simulink model "uz_pmsm_model_6LUT_pd"  (R2023b)
settings: Solver=FixedStepAuto  StartTime=0.0  StopTime=0.05  RelTol=1e-3
PreLoadFcn:
  | uz_pmsm_model_init_parameter
PostLoadFcn:
  | % Import the data from Excel for a lookup table
  | FluxMapData = readtable('C:\Users\Philipp\ultrazohm\ultrazohm_sw\ip_cores\uz_pmsm_model\FluxMapData_2023-05-26_13-07-57.csv');
  | % Row indices for lookup table
  | d_current_in_d_axis = FluxMapData(8:27,1:end);
  | % Column indices for lookup table
  | q_current_in_d_axis = FluxMapData(29:48,1:end);
  | % Output values for lookup table
  | d_Flux_d_axis = FluxMapData(50:69,1:end);
values from neighbouring files (symbols this model uses):
  ad1 = 7.2940    (= 7.294)    [LUT_approx_methode1_u_2b.m]    (also in LUT_approx_methode1_u_2b_alt.m; LUT_approx_methode2a.m = ad_1(1); LUT_approx_methode_2a_FEM.m = ad_1(1); LUT_approx_new.m = ad_1(1))
  ad2 = 0.0001    [LUT_approx_methode1_u_2b.m]    (also in LUT_approx_methode1_u_2b_alt.m; LUT_approx_methode2a.m = ad_1(2); LUT_approx_methode_2a_FEM.m = ad_1(2); LUT_approx_new.m = ad_1(2))
  ad3 = -15.5992    [LUT_approx_methode1_u_2b.m]    (also in LUT_approx_methode1_u_2b_alt.m; LUT_approx_methode2a.m = ad_1(3); LUT_approx_methode_2a_FEM.m = ad_1(3); LUT_approx_new.m = ad_1(3))
  ad4 = -186.4725    [LUT_approx_methode1_u_2b.m]    (also in LUT_approx_methode1_u_2b_alt.m; LUT_approx_methode2a.m = ad_3_6(1); LUT_approx_methode_2a_FEM.m = ad_3_6(1); LUT_approx_new.m = ad_3_6(1))
  ad5 = 187.4853    [LUT_approx_methode1_u_2b.m]    (also in LUT_approx_methode1_u_2b_alt.m; LUT_approx_methode2a.m = ad_3_6(2); LUT_approx_methode_2a_FEM.m = ad_3_6(2); LUT_approx_new.m = ad_3_6(2))
  ad6 = 0.0000    (= 0)    [LUT_approx_methode1_u_2b.m]    (also in LUT_approx_methode1_u_2b_alt.m; LUT_approx_methode2a.m = ad_3_6(3); LUT_approx_methode_2a_FEM.m = ad_3_6(3); LUT_approx_new.m = ad_3_6(3))
  aq1 = 0.0041    [LUT_approx_methode1_u_2b.m]    (also in LUT_approx_methode1_u_2b_alt.m; LUT_approx_methode2a.m = aq_1(1); LUT_approx_methode_2a_FEM.m = aq_1(1); LUT_approx_new.m = aq_1(1))
  aq2 = 0.2092    [LUT_approx_methode1_u_2b.m]    (also in LUT_approx_methode1_u_2b_alt.m; LUT_approx_methode2a.m = aq_1(2); LUT_approx_methode_2a_FEM.m = aq_1(2); LUT_approx_new.m = aq_1(2))
  aq3 = 0.0010    (= 0.001)    [LUT_approx_methode1_u_2b.m]    (also in LUT_approx_methode1_u_2b_alt.m; LUT_approx_methode2a.m = aq_1(3); LUT_approx_methode_2a_FEM.m = aq_1(3); LUT_approx_new.m = aq_1(3))
  aq4 = 28.4940    (= 28.494)    [LUT_approx_methode1_u_2b.m]    (also in LUT_approx_methode1_u_2b_alt.m; LUT_approx_methode2a.m = aq_3_6(1); LUT_approx_methode_2a_FEM.m = aq_3_6(1); LUT_approx_new.m = aq_3_6(1))
  aq5 = -24.2348    [LUT_approx_methode1_u_2b.m]    (also in LUT_approx_methode1_u_2b_alt.m; LUT_approx_methode2a.m = aq_3_6(2); LUT_approx_methode_2a_FEM.m = aq_3_6(2); LUT_approx_new.m = aq_3_6(2))
  aq6 = 0.0405    [LUT_approx_methode1_u_2b.m]    (also in LUT_approx_methode1_u_2b_alt.m; LUT_approx_methode2a.m = aq_3_6(3); LUT_approx_methode_2a_FEM.m = aq_3_6(3); LUT_approx_new.m = aq_3_6(3))
  d_current_d_Flux = FluxMapData{1,1:20}    [uz_pmsm_model_6LUT_pd_init_parameter.m]
  d_current_q_Flux = FluxMapData{66,1:20}    [uz_pmsm_model_6LUT_pd_init_parameter.m]
  entkopplung_dynamic = false    [uz_pmsm_model_6LUT_pd_init_parameter.m]
  entkopplung_linear = true    [uz_pmsm_model_6LUT_pd_init_parameter.m]
  entkopplung_static = false    [uz_pmsm_model_6LUT_pd_init_parameter.m]
  Fid1_Giq1 = ((1/2).*(aq3-aq6).*((q_current_set).^2))+((aq1./aq2).*log(cosh(aq2.*q_current_set)))-((aq4/aq5).*log(cosh(aq5.*q_current_set)))    [LUT_approx_methode2a.m]    (also in LUT_approx_methode_2a_FEM.m = (1/2).*(aq3-aq6).*((q_current_set).^2)+((aq1./aq2).*log(cosh; LUT_approx_new.m = (1/2)*(aq3-aq6)*((q_current_set).^2)+((aq1/aq2)*log(cosh(aq2; LUT_approximation_fitting.m = (1/2)*(aq3-aq6)*((iq1)^2)+((aq1/aq2)*log(cosh(aq2*iq1)))-((a)
  Fid2_Giq2 = ((ad1./ad2).*(log(cosh(ad2.*(d_current_set-ad3))))) - ((ad4./ad5).*(log(cosh(ad5.*(d_current_set-ad6)))))    [LUT_approx_methode2a.m]    (also in LUT_approx_methode_2a_FEM.m = ((ad1./ad2).*(log(cosh(ad2.*(d_current_set-ad3))))) - (((ad1)
  Flux_d = FluxMapData{43:62,1:20}'*(1e-3)    [uz_pmsm_model_6LUT_pd_init_parameter.m]
  Flux_q = FluxMapData{108:127,1:20}'*(1e-3)    [uz_pmsm_model_6LUT_pd_init_parameter.m]
  friction_coefficient = 0.001    [uz_pmsm_model_6LUT_pd_init_parameter.m]
  inertia = 0.000084    (= 8.4e-05)    [uz_pmsm_model_6LUT_pd_init_parameter.m]
  L_d = 0.00045    [uz_pmsm_model_6LUT_pd_init_parameter.m]
  L_q = 0.002    [uz_pmsm_model_6LUT_pd_init_parameter.m]
  parameter_nachfuerung = true    [uz_pmsm_model_6LUT_pd_init_parameter.m]
  polepair = 4    [uz_pmsm_model_6LUT_pd_init_parameter.m]
  praediktion_entkopplung_nonlinear = true    [uz_pmsm_model_6LUT_pd_init_parameter.m]
  psi_pm = 0.0194    [uz_pmsm_model_6LUT_pd_init_parameter.m]
  q_current_d_Flux = FluxMapData{22:41,1}    [uz_pmsm_model_6LUT_pd_init_parameter.m]
  q_current_q_Flux = FluxMapData{87:106,1}    [uz_pmsm_model_6LUT_pd_init_parameter.m]
  R_1 = 0.3    [uz_pmsm_model_6LUT_pd_init_parameter.m]
  simulate_mechanical = false    [uz_pmsm_model_6LUT_pd_init_parameter.m]
  simulate_nonlinear_modell = true    [uz_pmsm_model_6LUT_pd_init_parameter.m]
  simulate_open_loop = false    [uz_pmsm_model_6LUT_pd_init_parameter.m]
  static_friction_torque = 0.01    [uz_pmsm_model_6LUT_pd_init_parameter.m]
  tau_sum = 2*ts_regler    (= 8e-05)    [uz_pmsm_model_6LUT_pd_init_parameter.m]
  ts = 1/5e5    (= 2e-06)    [uz_pmsm_model_6LUT_pd_init_parameter.m]
  ts_regler = 1/25e3    (= 4e-05)    [uz_pmsm_model_6LUT_pd_init_parameter.m]
undefined symbols (not defined in the file or in its folder): Ki_Bo_d, Ki_Bo_q, Kp_Bo_d, Kp_Bo_q, Ldq
libraries: slpidlib x2
(part 1 of 2)
settings Model: DataTypeOverride=Off  Creator=ts  LastModifiedBy=Philipp
settings SolverCC: AlgebraicLoopSolver=TrustRegion  AutoInsertRateTranBlk=on
settings DataIOCC: LimitDataPoints=on  SaveOutput=off  SaveTime=off
settings OptimizationCC: BlockReduction=off  ConditionallyExecuteInputs=off  DefaultParameterBehavior=Inlined  LifeSpan=inf
settings DebuggingCC: AlgebraicLoopMsg=error  SingleTaskRateTransMsg=error  UnconnectedInputMsg=warning  UnconnectedOutputMsg=warning  UnconnectedLineMsg=warning  AllowSymbolicDim=off  StrictBusMsg=ErrorOnBusTreatedAsVector  SFUnexpectedBacktrackingDiag=warning  SFNoUnconditionalDefaultTransitionDiag=warning  SFExecutionAtInitializationDiag=none  ArithmeticOperatorsInVariantConditions=warning
settings HardwareCC: ProdBitPerPointer=32  ProdBitPerSizeT=32  ProdBitPerPtrDiffT=32  ProdLargestAtomicFloat=None  ProdIntDivRoundTo=Undefined  ProdEndianess=Unspecified  ProdWordSize=32  ProdHWDeviceType=ASIC/FPGA->ASIC/FPGA  ProdEqTarget=off
settings ModelReferenceCC: EnableRefExpFcnMdlSchedulingChecks=on
settings SFSimCC: SimUseLocalCustomCode=off  CustomCodeUndefinedFunction=UseInterfaceOnly
settings RTWCC: RTWUseLocalCustomCode=off  DLArmComputeVersion=19.05
settings CodeAppCC: StateflowObjectComments=on
settings GRTTargetCC: TargetLangStandard=C89/C90 (ANSI)
settings ConfigComp: CovScope=ReferencedModels  CovMetricSettings=dw  CovSaveCumulativeToWorkspaceVar=on  CovSaveSingleToWorkspaceVar=on  CovExternalEMLEnable=off  CovSFcnEnable=off

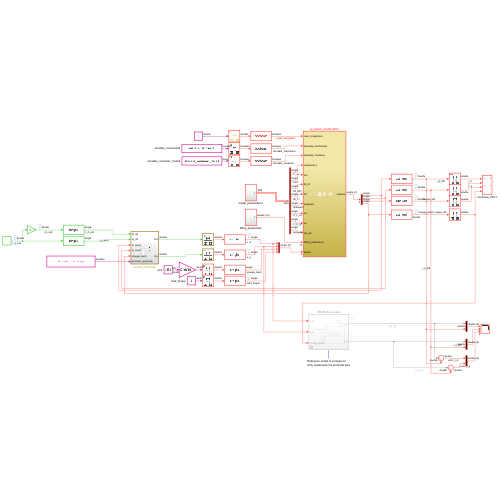
[thumbnail: Simulink's stored preview of the top-level diagram]
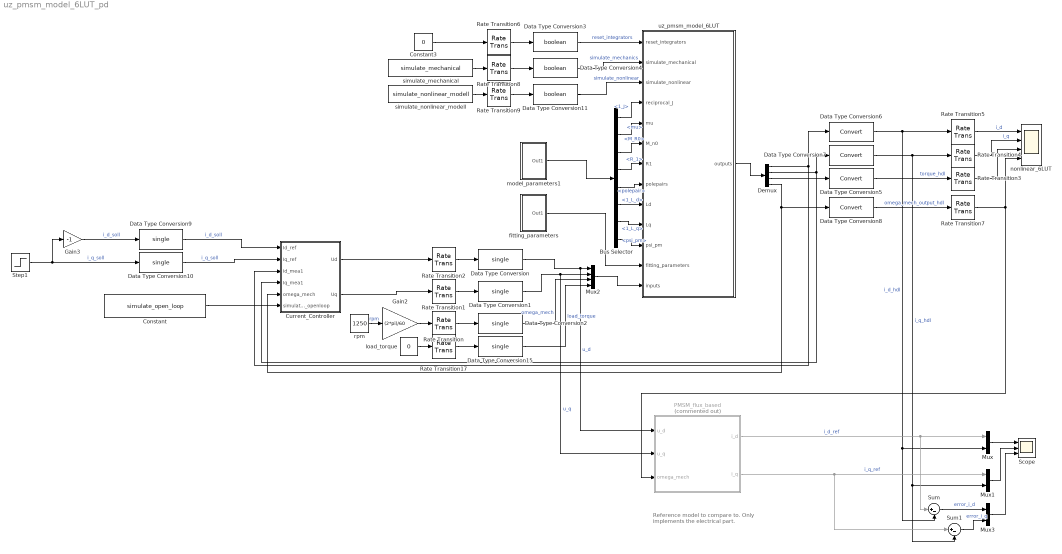
== system uz_pmsm_model_6LUT_pd ==
  note: Reference model to compare to.
      | Only implements the electrical part.
  Bus Selector : BusSelector  OutputSignals=1_J,mu,M_R0,R_1,polepair,1_L_d,1_L_q,psi_pm
  Constant : Constant  Value=simulate_open_loop
  Constant3 : Constant  Value=0
  Current_Controller : Subsystem
  Data Type Conversion{,1..2,9..10,15} (6 alike) : DataTypeConversion  OutDataTypeStr=single  SaturateOnIntegerOverflow=off  RndMeth=Floor
  Data Type Conversion11 : DataTypeConversion  OutDataTypeStr=boolean  SaturateOnIntegerOverflow=off  RndMeth=Floor
  Data Type Conversion3 : DataTypeConversion  OutDataTypeStr=boolean  SaturateOnIntegerOverflow=off  RndMeth=Floor
  Data Type Conversion4 : DataTypeConversion  OutDataTypeStr=boolean  SaturateOnIntegerOverflow=off  RndMeth=Floor
  Data Type Conversion{5..8} (4 alike) : DataTypeConversion  SaturateOnIntegerOverflow=off  RndMeth=Floor
  Demux : Demux
  Gain2 : Gain  Gain=(2*pi)/60
  Gain3 : Gain  Gain=-1
  Mux : Mux  Inputs=2
  Mux1 : Mux  Inputs=2
  Mux2 : Mux
  Mux3 : Mux  Inputs=2
  PMSM_flux_based : Subsystem  Commented=on
  Rate Transition{,1..2,6,8..9,17} (7 alike) : RateTransition  OutPortSampleTime=ts
  Rate Transition{3..5,7} (4 alike) : RateTransition
  Scope : Scope  NumInputPorts=3
  Step1 : Step  Time=0.025  After=5
  Sum : Sum  Inputs=|+-
  Sum1 : Sum  Inputs=|+-
  fitting_parameters : Subsystem
  load_torque : Constant  Value=0
  model_parameters1 : Subsystem
  nonlinear_6LUT : Scope  NumInputPorts=4
  rpm : Constant  Value=1250
  simulate_mechanical : Constant  Value=simulate_mechanical
  simulate_nonlinear_modell : Constant  Value=simulate_nonlinear_modell
  uz_pmsm_model_6LUT : Subsystem  TreatAsAtomicUnit=on
  wires:
  Rate Transition/1 -> Data Type Conversion2/1
  Rate Transition1/1 -> Data Type Conversion1/1
  Rate Transition2/1 -> Data Type Conversion/1
  Data Type Conversion6/1 -> Mux/2, Sum/2, Rate Transition5/1  "i_d_hdl"
  Data Type Conversion7/1 -> Rate Transition4/1, Mux1/2, Sum1/2  "i_q_hdl"
  Data Type Conversion5/1 -> Rate Transition3/1  "torque_hdl"
  Rate Transition4/1 -> nonlinear_6LUT/2  "i_q"
  Rate Transition5/1 -> nonlinear_6LUT/1  "i_d"
  Rate Transition3/1 -> nonlinear_6LUT/3
  Rate Transition6/1 -> Data Type Conversion3/1
  Constant3/1 -> Rate Transition6/1
  Rate Transition8/1 -> Data Type Conversion4/1
  simulate_mechanical/1 -> Rate Transition8/1
  Data Type Conversion3/1 -> uz_pmsm_model_6LUT/1(reset_integrators)  "reset_integrators"
  Data Type Conversion4/1 -> uz_pmsm_model_6LUT/2(simulate_mechanical)  "simulate_mechanics"
  load_torque/1 -> Rate Transition17/1
  Rate Transition17/1 -> Data Type Conversion15/1
  Mux/1 -> Scope/1
  Mux1/1 -> Scope/2
  PMSM_flux_based/2(i_q) -> Mux1/1, Sum1/1  "i_q_ref"
  PMSM_flux_based/1(i_d) -> Mux/1, Sum/1  "i_d_ref"
  Data Type Conversion8/1 -> Rate Transition7/1  "omega_mech_output_hdl"
  Rate Transition7/1 -> PMSM_flux_based/3(omega_mech), nonlinear_6LUT/4
  Bus Selector/1 -> uz_pmsm_model_6LUT/4(reciprocal_J)  "<1_J>"
  Bus Selector/2 -> uz_pmsm_model_6LUT/5(mu)  "<mu>"
  Bus Selector/3 -> uz_pmsm_model_6LUT/6(M_n0)  "<M_R0>"
  Bus Selector/4 -> uz_pmsm_model_6LUT/7(R1)  "<R_1>"
  Bus Selector/5 -> uz_pmsm_model_6LUT/8(polepairs)  "<polepair>"
  model_parameters1/1(Out1) -> Bus Selector/1
  Sum/1 -> Mux3/1  "error_i_d"
  Sum1/1 -> Mux3/2  "error_i_q"
  Mux3/1 -> Scope/3
  Step1/1 -> Gain3/1, Data Type Conversion10/1  "i_q_soll"
  Demux/3 -> Data Type Conversion5/1
  Gain3/1 -> Data Type Conversion9/1  "i_d_soll"
  Demux/1 -> Current_Controller/3(Id_mea1), Data Type Conversion6/1
  Demux/4 -> Current_Controller/5(omega_mech), Data Type Conversion8/1
  Demux/2 -> Current_Controller/4(Iq_mea1), Data Type Conversion7/1
  Data Type Conversion/1 -> PMSM_flux_based/1(u_d), Mux2/1  "u_d"
  Data Type Conversion1/1 -> PMSM_flux_based/2(u_q), Mux2/2  "u_q"
  Data Type Conversion15/1 -> Mux2/4  "load_torque"
  Data Type Conversion2/1 -> Mux2/3  "omega_mech"
  Mux2/1 -> uz_pmsm_model_6LUT/13(inputs)
  uz_pmsm_model_6LUT/1(outputs) -> Demux/1
  Data Type Conversion9/1 -> Current_Controller/1(Id_ref)  "i_d_soll"
  Data Type Conversion10/1 -> Current_Controller/2(Iq_ref)  "i_q_soll"
  Current_Controller/1(Ud) -> Rate Transition2/1
  Current_Controller/2(Uq) -> Rate Transition1/1
  Gain2/1 -> Rate Transition/1
  Constant/1 -> Current_Controller/6(simulate_openloop)
  rpm/1 -> Gain2/1  "rpm"
  simulate_nonlinear_modell/1 -> Rate Transition9/1
  Rate Transition9/1 -> Data Type Conversion11/1
  Bus Selector/6 -> uz_pmsm_model_6LUT/9(Ld)  "<1_L_d>"
  Bus Selector/7 -> uz_pmsm_model_6LUT/10(Lq)  "<1_L_q>"
  Bus Selector/8 -> uz_pmsm_model_6LUT/11(psi_pm)  "<psi_pm>"
  Data Type Conversion11/1 -> uz_pmsm_model_6LUT/3(simulate_nonlinear)  "simulate_nonlinear"
  fitting_parameters/1(Out1) -> uz_pmsm_model_6LUT/12(fitting_parameters)

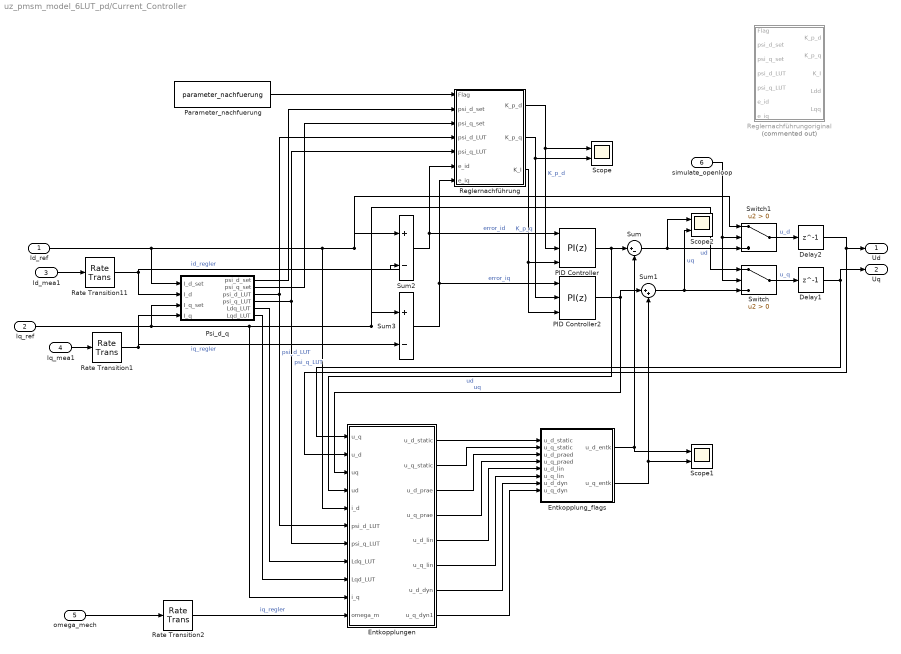
== system uz_pmsm_model_6LUT_pd/Current_Controller ==
  Id_ref : Inport
  Iq_ref : Inport  Port=2
  Id_mea1 : Inport  Port=3
  Iq_mea1 : Inport  Port=4
  omega_mech : Inport  Port=5
  simulate_openloop : Inport  Port=6
  Delay1 : Delay  DelayLength=1
  Delay2 : Delay  DelayLength=1
  Entkopplung_flags : Subsystem
  Entkopplungen : Subsystem
  PID Controller : slpidlib/PID Controller  Controller=PI  Form=Parallel  TimeDomain=Discrete-time  UseExternalTs=off  SampleTime=-1  IntegratorMethod=Forward Euler  FilterMethod=Forward Euler  ControllerParametersSource=external  P=Kp_Bo_d  I=Ki_Bo_d  UseKiTs=off  D=0  N=100  UseFilter=on  TunerSelectOption=Transfer Function Based (PID Tuner App)  InitialConditionSource=internal  InitialConditionForIntegrator=0  InitialConditionForFilter=0  DifferentiatorICPrevScaledInput=0  ExternalReset=none  TrackingMode=off  Kt=1  LimitOutput=off  SatLimitsSource=internal  UpperSaturationLimit=48  LowerSaturationLimit=-48  LinearizeAsGain=off  AntiWindupMode=clamping  Kb=1  LimitIntegrator=off  UpperIntegratorSaturationLimit=48  LowerIntegratorSaturationLimit=-48  POutMin=[]  POutMax=[]  IOutMin=[]  IOutMax=[]  DOutMin=[]  DOutMax=[]  NOutMin=[]  NOutMax=[]  SumOutMin=[]  SumOutMax=[]  SaturationOutMin=[]  SaturationOutMax=[]  PParamMin=[]  PParamMax=[]  IParamMin=[]  IParamMax=[]  DParamMin=[]  DParamMax=[]  NParamMin=[]  NParamMax=[]  KbParamMin=[]  KbParamMax=[]  KtParamMin=[]  KtParamMax=[]  KbOutMin=[]  KbOutMax=[]  KtOutMin=[]  KtOutMax=[]  IntegratorOutMin=[]  IntegratorOutMax=[]  FilterOutMin=[]  FilterOutMax=[]  SumI1OutMin=[]  SumI1OutMax=[]  SumI2OutMin=[]  SumI2OutMax=[]  SumI3OutMin=[]  SumI3OutMax=[]  SumI4OutMin=[]  SumI4OutMax=[]  SumDOutMin=[]  SumDOutMax=[]  DifferentiatorOutMin=[]  DifferentiatorOutMax=[]  FilterDiffOutCoefMin=[]  FilterDiffOutCoefMax=[]  ReciprocalOutMin=[]  ReciprocalOutMax=[]  SumDenOutMin=[]  SumDenOutMax=[]  SumNumOutMin=[]  SumNumOutMax=[]  DivideOutMin=[]  DivideOutMax=[]  UdiffTsProdOutMin=[]  UdiffTsProdOutMax=[]  NTsProdOutMin=[]  NTsProdOutMax=[]  UintegralTsProdOutMin=[]  UintegralTsProdOutMax=[]  UngainTsProdOutMin=[]  UngainTsProdOutMax=[]  ClampingZeroOutDataTypeStr=Inherit: Inherit via back propagation  ClampingZeroOutMin=[]  ClampingZeroOutMax=[]  FilterDenConstantOutDataTypeStr=Inherit: Inherit via back propagation  FilterDenConstantOutMin=[]  FilterDenConstantOutMax=[]  PCopyOutDataTypeStr=Inherit: Inherit via back propagation  PCopyOutMin=[]  PCopyOutMax=[]  NCopyOutDataTypeStr=Inherit: Inherit via back propagation  NCopyOutMin=[]  NCopyOutMax=[]  IntegratorContinuousStateAttributes=''  IntegratorStateMustResolveToSignalObject=off  IntegratorRTWStateStorageClass=Auto  FilterContinuousStateAttributes=''  FilterStateMustResolveToSignalObject=off  FilterRTWStateStorageClass=Auto  ParallelPVariant=ExternalParameters  IdealPVariant=Disabled  IVariant=ExternalParameters  DVariant=Disabled  IntegratorVariant=Discrete  SatVariant=Disabled  AWVariant=Passthrough  PCopyVariant=Disabled  TRVariant=Disabled  FdbkBlocksVariant=Forward  IdealPFdbkVariant=Disabled  SatFdbkVariant=Disabled  DerivativeFilterVariant=Disabled  NVariant=Disabled  NCopyVariant=Disabled_SignalSpec  FilterICVariant=Disabled  IntegratorICVariant=InternalICs  ExternalResetVariant=Disabled  TRSumVariant=Passthrough  SumFdbkVariant=Disabled  SumVariant=Sum_PI  TsampFilterVariant=InternalTs  TsampNgainVariant=Passthrough  TsampIntegralVariant=Disabled_SignalSpec  ExternalSaturationOutDataTypeStr=Inherit: Same as second input
  PID Controller2 : slpidlib/PID Controller  Controller=PI  Form=Parallel  TimeDomain=Discrete-time  UseExternalTs=off  SampleTime=-1  IntegratorMethod=Forward Euler  FilterMethod=Forward Euler  ControllerParametersSource=external  P=Kp_Bo_q  I=Ki_Bo_q  UseKiTs=off  D=0  N=100  UseFilter=on  TunerSelectOption=Transfer Function Based (PID Tuner App)  InitialConditionSource=internal  InitialConditionForIntegrator=0  InitialConditionForFilter=0  DifferentiatorICPrevScaledInput=0  ExternalReset=none  TrackingMode=off  Kt=1  LimitOutput=off  SatLimitsSource=internal  UpperSaturationLimit=48  LowerSaturationLimit=-48  LinearizeAsGain=off  AntiWindupMode=clamping  Kb=1  LimitIntegrator=off  UpperIntegratorSaturationLimit=48  LowerIntegratorSaturationLimit=-48  POutMin=[]  POutMax=[]  IOutMin=[]  IOutMax=[]  DOutMin=[]  DOutMax=[]  NOutMin=[]  NOutMax=[]  SumOutMin=[]  SumOutMax=[]  SaturationOutMin=[]  SaturationOutMax=[]  PParamMin=[]  PParamMax=[]  IParamMin=[]  IParamMax=[]  DParamMin=[]  DParamMax=[]  NParamMin=[]  NParamMax=[]  KbParamMin=[]  KbParamMax=[]  KtParamMin=[]  KtParamMax=[]  KbOutMin=[]  KbOutMax=[]  KtOutMin=[]  KtOutMax=[]  IntegratorOutMin=[]  IntegratorOutMax=[]  FilterOutMin=[]  FilterOutMax=[]  SumI1OutMin=[]  SumI1OutMax=[]  SumI2OutMin=[]  SumI2OutMax=[]  SumI3OutMin=[]  SumI3OutMax=[]  SumI4OutMin=[]  SumI4OutMax=[]  SumDOutMin=[]  SumDOutMax=[]  DifferentiatorOutMin=[]  DifferentiatorOutMax=[]  FilterDiffOutCoefMin=[]  FilterDiffOutCoefMax=[]  ReciprocalOutMin=[]  ReciprocalOutMax=[]  SumDenOutMin=[]  SumDenOutMax=[]  SumNumOutMin=[]  SumNumOutMax=[]  DivideOutMin=[]  DivideOutMax=[]  UdiffTsProdOutMin=[]  UdiffTsProdOutMax=[]  NTsProdOutMin=[]  NTsProdOutMax=[]  UintegralTsProdOutMin=[]  UintegralTsProdOutMax=[]  UngainTsProdOutMin=[]  UngainTsProdOutMax=[]  ClampingZeroOutDataTypeStr=Inherit: Inherit via back propagation  ClampingZeroOutMin=[]  ClampingZeroOutMax=[]  FilterDenConstantOutDataTypeStr=Inherit: Inherit via back propagation  FilterDenConstantOutMin=[]  FilterDenConstantOutMax=[]  PCopyOutDataTypeStr=Inherit: Inherit via back propagation  PCopyOutMin=[]  PCopyOutMax=[]  NCopyOutDataTypeStr=Inherit: Inherit via back propagation  NCopyOutMin=[]  NCopyOutMax=[]  IntegratorContinuousStateAttributes=''  IntegratorStateMustResolveToSignalObject=off  IntegratorRTWStateStorageClass=Auto  FilterContinuousStateAttributes=''  FilterStateMustResolveToSignalObject=off  FilterRTWStateStorageClass=Auto  ParallelPVariant=ExternalParameters  IdealPVariant=Disabled  IVariant=ExternalParameters  DVariant=Disabled  IntegratorVariant=Discrete  SatVariant=Disabled  AWVariant=Passthrough  PCopyVariant=Disabled  TRVariant=Disabled  FdbkBlocksVariant=Forward  IdealPFdbkVariant=Disabled  SatFdbkVariant=Disabled  DerivativeFilterVariant=Disabled  NVariant=Disabled  NCopyVariant=Disabled_SignalSpec  FilterICVariant=Disabled  IntegratorICVariant=InternalICs  ExternalResetVariant=Disabled  TRSumVariant=Passthrough  SumFdbkVariant=Disabled  SumVariant=Sum_PI  TsampFilterVariant=InternalTs  TsampNgainVariant=Passthrough  TsampIntegralVariant=Disabled_SignalSpec  ExternalSaturationOutDataTypeStr=Inherit: Same as second input
  Parameter_nachfuerung : Constant  Value=parameter_nachfuerung
  Psi_d_q : Subsystem
  Rate Transition1 : RateTransition  OutPortSampleTime=ts_regler
  Rate Transition11 : RateTransition  OutPortSampleTime=ts_regler
  Rate Transition2 : RateTransition  OutPortSampleTime=ts_regler
  Reglernachführung : Subsystem
  Reglernachführungoriginal : Subsystem  Commented=on
  Scope : Scope  NumInputPorts=2
  Scope1 : Scope  NumInputPorts=2
  Scope2 : Scope  NumInputPorts=2
  Sum : Sum  Inputs=|+-
  Sum1 : Sum  Inputs=|++
  Sum2 : Sum  Inputs=|+-
  Sum3 : Sum  Inputs=|+-
  Switch : Switch  Criteria=u2 > Threshold  SaturateOnIntegerOverflow=off  InputSameDT=off
  Switch1 : Switch  Criteria=u2 > Threshold  SaturateOnIntegerOverflow=off  InputSameDT=off
  Ud : Outport
  Uq : Outport  Port=2
  wires:
  Sum3/1 -> Reglernachführung/7(e_iq), PID Controller2/1  "error_iq"
  Sum2/1 -> PID Controller/1, Reglernachführung/6(e_id)  "error_id"
  Sum/1 -> Scope2/1, Switch1/3  "ud"
  PID Controller/1 -> Entkopplungen/4(ud), Sum/1  "ud"
  PID Controller2/1 -> Sum1/1, Entkopplungen/3(uq)  "uq"
  Sum1/1 -> Scope2/2, Switch/3  "uq"
  Iq_ref/1 -> Entkopplungen/10(i_q), Sum3/1, Switch/1, Psi_d_q/3(I_q_set)
  Id_ref/1 -> Psi_d_q/1(I_d_set), Entkopplungen/5(i_d), Sum2/1, Switch1/1
  Switch/1 -> Delay1/1  "u_q"
  Switch1/1 -> Delay2/1  "u_d"
  simulate_openloop/1 -> Switch/2, Switch1/2
  Reglernachführung/1(K_p_d) -> PID Controller/2, Scope/1  "K_p_d"
  Reglernachführung/2(K_p_q) -> PID Controller2/2, Scope/2  "K_p_q"
  Reglernachführung/3(K_I) -> PID Controller2/3, PID Controller/3
  Id_mea1/1 -> Rate Transition11/1
  Iq_mea1/1 -> Rate Transition1/1
  Psi_d_q/3(psi_d_LUT) -> Entkopplungen/6(psi_d_LUT), Reglernachführung/4(psi_d_LUT)  "psi_d_LUT"
  Psi_d_q/4(psi_q_LUT) -> Entkopplungen/7(psi_q_LUT), Reglernachführung/5(psi_q_LUT)  "psi_q_LUT"
  Parameter_nachfuerung/1 -> Reglernachführung/1(Flag)
  Psi_d_q/1(psi_d_set) -> Reglernachführung/2(psi_d_set)
  Psi_d_q/2(psi_q_set) -> Reglernachführung/3(psi_q_set)
  omega_mech/1 -> Rate Transition2/1
  Entkopplungen/1(u_d_static) -> Entkopplung_flags/1(u_d_static)
  Entkopplungen/2(u_q_static) -> Entkopplung_flags/2(u_q_static)
  Entkopplungen/3(u_d_prae) -> Entkopplung_flags/3(u_d_praed)
  Entkopplungen/4(u_q_prae) -> Entkopplung_flags/4(u_q_praed)
  Entkopplungen/5(u_d_lin) -> Entkopplung_flags/5(u_d_lin)
  Entkopplungen/6(u_q_lin) -> Entkopplung_flags/6(u_q_lin)
  Entkopplung_flags/1(u_d_entk) -> Scope1/1, Sum/2
  Entkopplung_flags/2(u_q_entk) -> Scope1/2, Sum1/2
  Rate Transition11/1 -> Sum2/2, Psi_d_q/2(I_d)  "id_regler"
  Rate Transition1/1 -> Sum3/2, Psi_d_q/4(I_q)  "iq_regler"
  Rate Transition2/1 -> Entkopplungen/11(omega_m)  "iq_regler"
  Delay2/1 -> Ud/1, Entkopplungen/2(u_d)
  Delay1/1 -> Uq/1, Entkopplungen/1(u_q)
  Entkopplungen/7(u_d_dyn) -> Entkopplung_flags/7(u_d_dyn)
  Entkopplungen/8(u_q_dyn1) -> Entkopplung_flags/8(u_q_dyn)
  Psi_d_q/5(Ldq_LUT) -> Entkopplungen/8(Ldq_LUT)
  Psi_d_q/6(Lqd_LUT) -> Entkopplungen/9(Lqd_LUT)

== system uz_pmsm_model_6LUT_pd/PMSM_flux_based ==
  u_d : Inport
  u_q : Inport  Port=2
  omega_mech : Inport  Port=3
  Constant : Constant  Value=psi_pm
  Gain : Gain  Gain=R_1
  Gain1 : Gain  Gain=1/L_d
  Gain2 : Gain  Gain=R_1
  Gain3 : Gain  Gain=1/L_q
  Gain6 : Gain  Gain=polepair
  Integrator : Integrator
  Integrator1 : Integrator
  Product : Product
  Product1 : Product
  Sum : Sum  Inputs=-++
  Sum1 : Sum  Inputs=-+-
  Sum2 : Sum  Inputs=+-
  i_d : Outport
  i_q : Outport  Port=2
  wires:
  u_d/1 -> Sum/2
  u_q/1 -> Sum1/2
  Sum/1 -> Integrator/1
  Gain/1 -> Sum/1
  Integrator/1 -> Product1/2, Sum2/1
  Constant/1 -> Sum2/2
  Sum2/1 -> Gain1/1
  Gain1/1 -> Gain/1, i_d/1
  Gain6/1 -> Product1/1, Product/1
  Product/1 -> Sum/3
  Integrator1/1 -> Gain3/1, Product/2
  Product1/1 -> Sum1/3
  Sum1/1 -> Integrator1/1
  Gain2/1 -> Sum1/1
  Gain3/1 -> i_q/1, Gain2/1
  omega_mech/1 -> Gain6/1

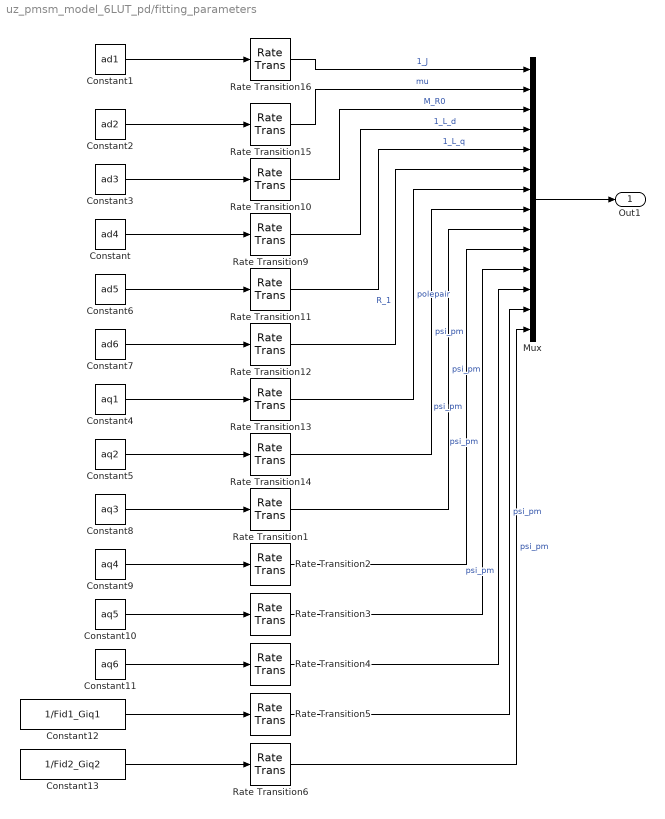
== system uz_pmsm_model_6LUT_pd/fitting_parameters ==
  Constant : Constant  Value=ad4
  Constant1 : Constant  Value=ad1
  Constant10 : Constant  Value=aq5
  Constant11 : Constant  Value=aq6
  Constant12 : Constant  Value=1/Fid1_Giq1
  Constant13 : Constant  Value=1/Fid2_Giq2
  Constant2 : Constant  Value=ad2
  Constant3 : Constant  Value=ad3
  Constant4 : Constant  Value=aq1
  Constant5 : Constant  Value=aq2
  Constant6 : Constant  Value=ad5
  Constant7 : Constant  Value=ad6
  Constant8 : Constant  Value=aq3
  Constant9 : Constant  Value=aq4
  Mux : Mux  Inputs=14
  Rate Transition{1..6,9..16} (14 alike) : RateTransition  OutPortSampleTime=ts
  Out1 : Outport
  wires:
  Constant1/1 -> Rate Transition16/1
  Constant/1 -> Rate Transition9/1
  Rate Transition10/1 -> Mux/3  "M_R0"
  Rate Transition14/1 -> Mux/8  "psi_pm"
  Constant3/1 -> Rate Transition10/1
  Rate Transition12/1 -> Mux/6  "R_1"
  Rate Transition16/1 -> Mux/1  "1_J"
  Rate Transition13/1 -> Mux/7  "polepair"
  Mux/1 -> Out1/1
  Constant5/1 -> Rate Transition14/1
  Constant7/1 -> Rate Transition12/1
  Rate Transition15/1 -> Mux/2  "mu"
  Rate Transition9/1 -> Mux/4  "1_L_d"
  Constant6/1 -> Rate Transition11/1
  Constant4/1 -> Rate Transition13/1
  Rate Transition11/1 -> Mux/5  "1_L_q"
  Constant2/1 -> Rate Transition15/1
  Rate Transition1/1 -> Mux/9  "psi_pm"
  Constant8/1 -> Rate Transition1/1
  Rate Transition2/1 -> Mux/10  "psi_pm"
  Constant9/1 -> Rate Transition2/1
  Rate Transition3/1 -> Mux/11  "psi_pm"
  Constant10/1 -> Rate Transition3/1
  Rate Transition4/1 -> Mux/12  "psi_pm"
  Constant11/1 -> Rate Transition4/1
  Rate Transition5/1 -> Mux/13  "psi_pm"
  Constant12/1 -> Rate Transition5/1
  Constant13/1 -> Rate Transition6/1
  Rate Transition6/1 -> Mux/14  "psi_pm"

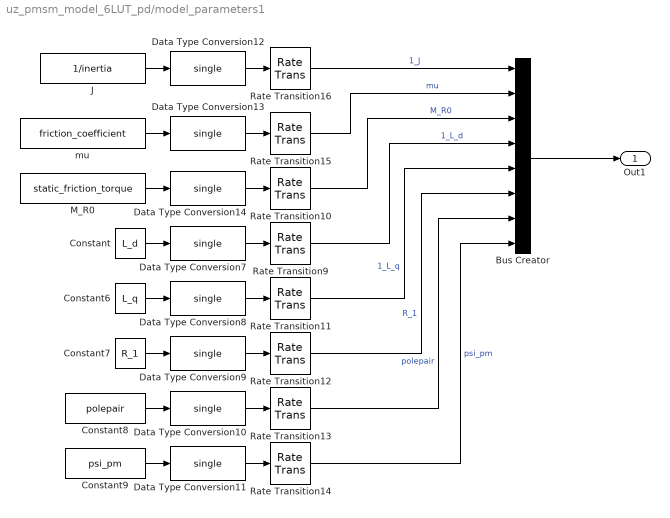
== system uz_pmsm_model_6LUT_pd/model_parameters1 ==
  Bus Creator : BusCreator  Inputs=8
  Constant : Constant  Value=L_d
  Constant6 : Constant  Value=L_q
  Constant7 : Constant  Value=R_1
  Constant8 : Constant  Value=polepair
  Constant9 : Constant  Value=psi_pm
  Data Type Conversion{7..14} (8 alike) : DataTypeConversion  OutDataTypeStr=single  SaturateOnIntegerOverflow=off  RndMeth=Floor
  J : Constant  Value=1/inertia
  M_R0 : Constant  Value=static_friction_torque
  Rate Transition{9..16} (8 alike) : RateTransition  OutPortSampleTime=ts
  mu : Constant  Value=friction_coefficient
  Out1 : Outport
  wires:
  Data Type Conversion12/1 -> Rate Transition16/1
  Data Type Conversion7/1 -> Rate Transition9/1
  Rate Transition10/1 -> Bus Creator/3  "M_R0"
  Rate Transition14/1 -> Bus Creator/8  "psi_pm"
  Data Type Conversion14/1 -> Rate Transition10/1
  Rate Transition12/1 -> Bus Creator/6  "R_1"
  Rate Transition16/1 -> Bus Creator/1  "1_J"
  Rate Transition13/1 -> Bus Creator/7  "polepair"
  Bus Creator/1 -> Out1/1
  Data Type Conversion11/1 -> Rate Transition14/1
  Constant8/1 -> Data Type Conversion10/1
  Data Type Conversion9/1 -> Rate Transition12/1
  Rate Transition15/1 -> Bus Creator/2  "mu"
  Constant6/1 -> Data Type Conversion8/1
  Rate Transition9/1 -> Bus Creator/4  "1_L_d"
  J/1 -> Data Type Conversion12/1
  Data Type Conversion8/1 -> Rate Transition11/1
  Data Type Conversion10/1 -> Rate Transition13/1
  mu/1 -> Data Type Conversion13/1
  M_R0/1 -> Data Type Conversion14/1
  Rate Transition11/1 -> Bus Creator/5  "1_L_q"
  Data Type Conversion13/1 -> Rate Transition15/1
  Constant7/1 -> Data Type Conversion9/1
  Constant9/1 -> Data Type Conversion11/1
  Constant/1 -> Data Type Conversion7/1

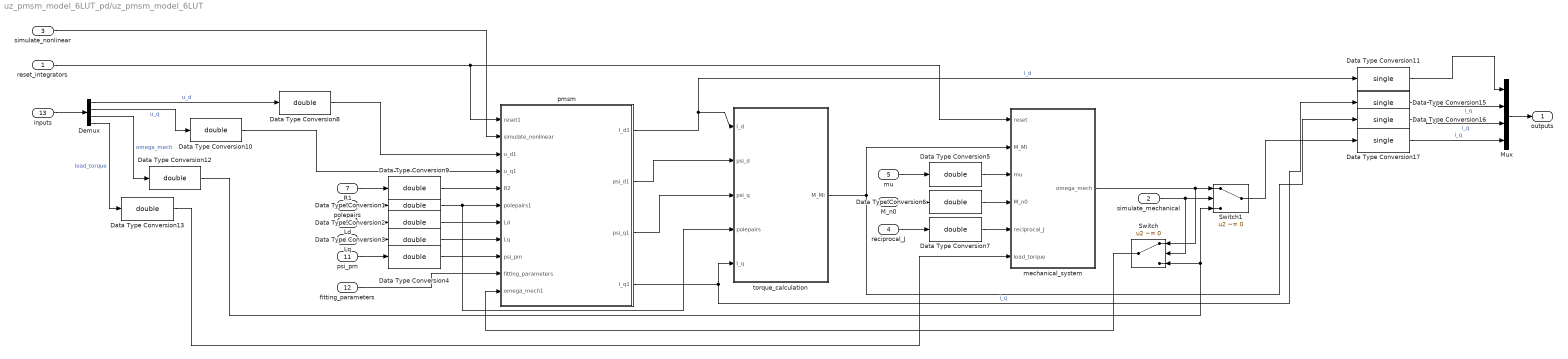
== system uz_pmsm_model_6LUT_pd/uz_pmsm_model_6LUT ==
  reset_integrators : Inport
  simulate_mechanical : Inport  Port=2
  simulate_nonlinear : Inport  Port=3
  reciprocal_J : Inport  Port=4
  mu : Inport  Port=5
  M_n0 : Inport  Port=6
  R1 : Inport  Port=7
  polepairs : Inport  Port=8
  Ld : Inport  Port=9
  Lq : Inport  Port=10
  psi_pm : Inport  Port=11
  fitting_parameters : Inport  Port=12
  inputs : Inport  Port=13
  Data Type Conversion{1..10,12..13} (12 alike) : DataTypeConversion  OutDataTypeStr=double  RndMeth=Nearest  SaturateOnIntegerOverflow=off
  Data Type Conversion{11,15..17} (4 alike) : DataTypeConversion  OutDataTypeStr=single  RndMeth=Nearest  SaturateOnIntegerOverflow=off
  Demux : Demux
  Mux : Mux
  Switch : Switch  Criteria=u2 ~= 0  SaturateOnIntegerOverflow=off  InputSameDT=off
  Switch1 : Switch  Criteria=u2 ~= 0  SaturateOnIntegerOverflow=off  InputSameDT=off
  mechanical_system : Subsystem
  pmsm : Subsystem
  torque_calculation : Subsystem
  outputs : Outport
  wires:
  reset_integrators/1 -> pmsm/1(reset1), mechanical_system/1(reset)
  Demux/3 -> Data Type Conversion12/1  "omega_mech"
  Switch/1 -> pmsm/11(omega_mech1)
  pmsm/2(psi_d1) -> torque_calculation/2(psi_d)
  Demux/4 -> Data Type Conversion13/1  "load_torque"
  Switch1/1 -> Data Type Conversion17/1
  R1/1 -> Data Type Conversion9/1
  pmsm/3(psi_q1) -> torque_calculation/3(psi_q)
  polepairs/1 -> Data Type Conversion1/1
  Demux/1 -> Data Type Conversion8/1  "u_d"
  mu/1 -> Data Type Conversion5/1
  simulate_mechanical/1 -> Switch1/2, Switch/2
  reciprocal_J/1 -> Data Type Conversion7/1
  torque_calculation/1(M_Mi) -> mechanical_system/2(M_Mi), Data Type Conversion16/1
  M_n0/1 -> Data Type Conversion6/1
  Demux/2 -> Data Type Conversion10/1  "u_q"
  mechanical_system/1(omega_mech) -> Switch/1, Switch1/1
  pmsm/4(I_q1) -> torque_calculation/5(I_q), Data Type Conversion15/1  "i_q"
  pmsm/1(I_d1) -> Data Type Conversion11/1, torque_calculation/1(I_d)  "i_d"
  Data Type Conversion17/1 -> Mux/4  "i_q"
  Data Type Conversion16/1 -> Mux/3  "i_q"
  Data Type Conversion15/1 -> Mux/2  "i_q"
  Data Type Conversion11/1 -> Mux/1
  inputs/1 -> Demux/1
  Mux/1 -> outputs/1
  psi_pm/1 -> Data Type Conversion4/1
  Lq/1 -> Data Type Conversion3/1
  Ld/1 -> Data Type Conversion2/1
  simulate_nonlinear/1 -> pmsm/2(simulate_nonlinear)
  fitting_parameters/1 -> pmsm/10(fitting_parameters)
  Data Type Conversion9/1 -> pmsm/5(R2)
  Data Type Conversion1/1 -> torque_calculation/4(polepairs), pmsm/6(polepairs1)
  Data Type Conversion2/1 -> pmsm/7(Ld)
  Data Type Conversion3/1 -> pmsm/8(Lq)
  Data Type Conversion4/1 -> pmsm/9(psi_pm)
  Data Type Conversion5/1 -> mechanical_system/3(mu)
  Data Type Conversion6/1 -> mechanical_system/4(M_n0)
  Data Type Conversion7/1 -> mechanical_system/5(reciprocal_J)
  Data Type Conversion8/1 -> pmsm/3(u_d1)
  Data Type Conversion10/1 -> pmsm/4(u_q1)
  Data Type Conversion12/1 -> Switch1/3, Switch/3
  Data Type Conversion13/1 -> mechanical_system/6(load_torque)

== system uz_pmsm_model_6LUT_pd/Current_Controller/Entkopplung_flags ==
  u_d_static : Inport
  u_q_static : Inport  Port=2
  u_d_praed : Inport  Port=3
  u_q_praed : Inport  Port=4
  u_d_lin : Inport  Port=5
  u_q_lin : Inport  Port=6
  u_d_dyn : Inport  Port=7
  u_q_dyn : Inport  Port=8
  0 : Constant  Value=0
  Switch{1..8} (8 alike) : Switch  Criteria=u2 > Threshold  SaturateOnIntegerOverflow=off  InputSameDT=off
  entkopplung_dynamic : Constant  Value=entkopplung_dynamic
  entkopplung_linear : Constant  Value=entkopplung_linear
  entkopplung_preadiktion : Constant  Value=praediktion_entkopplung_nonlinear
  entkopplung_static : Constant  Value=entkopplung_static
  u_d_entk : Outport
  u_q_entk : Outport  Port=2
  wires:
  Switch3/1 -> u_d_entk/1
  Switch4/1 -> Switch2/3
  entkopplung_preadiktion/1 -> Switch2/2, Switch3/2
  Switch1/1 -> Switch3/3
  u_d_praed/1 -> Switch3/1
  Switch2/1 -> u_q_entk/1
  u_q_praed/1 -> Switch2/1
  entkopplung_static/1 -> Switch4/2, Switch1/2
  u_d_static/1 -> Switch1/1
  u_d_lin/1 -> Switch5/1
  Switch5/1 -> Switch1/3
  entkopplung_linear/1 -> Switch6/2, Switch5/2
  entkopplung_dynamic/1 -> Switch8/2, Switch7/2
  0/1 -> Switch8/3, Switch7/3
  Switch6/1 -> Switch4/3
  u_q_static/1 -> Switch4/1
  u_q_lin/1 -> Switch6/1
  u_d_dyn/1 -> Switch7/1
  Switch8/1 -> Switch6/3
  u_q_dyn/1 -> Switch8/1
  Switch7/1 -> Switch5/3

== system uz_pmsm_model_6LUT_pd/Current_Controller/Entkopplungen ==
  u_q : Inport
  u_d : Inport  Port=2
  uq : Inport  Port=3
  ud : Inport  Port=4
  i_d : Inport  Port=5
  psi_d_LUT : Inport  Port=6
  psi_q_LUT : Inport  Port=7
  Ldq_LUT : Inport  Port=8
  Lqd_LUT : Inport  Port=9
  i_q : Inport  Port=10
  omega_m : Inport  Port=11
  Lineare_Entkopplung : Subsystem
  decoupling_praediktion : Subsystem
  dynamic_nonlinear_entkopplung1 : Subsystem
  static_nonlinear_entkopplung : Subsystem
  u_d_static : Outport
  u_q_static : Outport  Port=2
  u_d_prae : Outport  Port=3
  u_q_prae : Outport  Port=4
  u_d_lin : Outport  Port=5
  u_q_lin : Outport  Port=6
  u_d_dyn : Outport  Port=7
  u_q_dyn1 : Outport  Port=8
  wires:
  psi_d_LUT/1 -> static_nonlinear_entkopplung/1(psi_d), dynamic_nonlinear_entkopplung1/3(psi_d), decoupling_praediktion/9(psi_d)
  omega_m/1 -> dynamic_nonlinear_entkopplung1/7(omega_m), Lineare_Entkopplung/3(omega_m), static_nonlinear_entkopplung/3(omega_m), decoupling_praediktion/5(omega_m)
  psi_q_LUT/1 -> dynamic_nonlinear_entkopplung1/4(psi_q), decoupling_praediktion/8(psi_q), static_nonlinear_entkopplung/2(psi_q)
  u_q/1 -> decoupling_praediktion/4(u_q_1)
  i_d/1 -> dynamic_nonlinear_entkopplung1/1(i_d), Lineare_Entkopplung/1(i_d), decoupling_praediktion/1(i_d)
  i_q/1 -> dynamic_nonlinear_entkopplung1/2(i_q), Lineare_Entkopplung/2(i_q), decoupling_praediktion/3(i_q)
  ud/1 -> decoupling_praediktion/6(u_d_k)
  uq/1 -> decoupling_praediktion/7(u_q_k)
  u_d/1 -> decoupling_praediktion/2(u_d_1)
  static_nonlinear_entkopplung/1(u_d) -> u_d_static/1
  Lineare_Entkopplung/1(u_d) -> u_d_lin/1
  static_nonlinear_entkopplung/2(u_q) -> u_q_static/1
  decoupling_praediktion/1(u_d_entk) -> u_d_prae/1
  Lineare_Entkopplung/2(u_q) -> u_q_lin/1
  decoupling_praediktion/2(u_q_entk) -> u_q_prae/1
  dynamic_nonlinear_entkopplung1/1(u_d) -> u_d_dyn/1
  dynamic_nonlinear_entkopplung1/2(u_q) -> u_q_dyn1/1
  Ldq_LUT/1 -> dynamic_nonlinear_entkopplung1/5(Ldq_LUT)
  Lqd_LUT/1 -> dynamic_nonlinear_entkopplung1/6(Lqd_LUT)

== system uz_pmsm_model_6LUT_pd/Current_Controller/Psi_d_q ==
  I_d_set : Inport
  I_d : Inport  Port=2
  I_q_set : Inport  Port=3
  I_q : Inport  Port=4
  Flux_d Lookup Table : Lookup_n-D  BreakpointsForDimension1=d_current_d_Flux  BreakpointsForDimension2=q_current_d_Flux  BreakpointsForDimension3=[5, 7]  Table=Flux_d  InternalRulePriority=Speed  RndMeth=Simplest
      settings: InputPortMap=u0,u1
  Flux_d Lookup Table1 : Lookup_n-D  BreakpointsForDimension1=d_current_d_Flux  BreakpointsForDimension2=q_current_d_Flux  BreakpointsForDimension3=[5, 7]  Table=Flux_d  InternalRulePriority=Speed  RndMeth=Simplest
      settings: InputPortMap=u0,u1
  Flux_q Lookup Table1 : Lookup_n-D  BreakpointsForDimension1=d_current_q_Flux  BreakpointsForDimension2=q_current_q_Flux  BreakpointsForDimension3=[5, 7]  Table=Flux_q  InternalRulePriority=Speed  RndMeth=Simplest
      settings: InputPortMap=u0,u1
  Flux_q Lookup Table2 : Lookup_n-D  BreakpointsForDimension1=d_current_q_Flux  BreakpointsForDimension2=q_current_q_Flux  BreakpointsForDimension3=[5, 7]  Table=Flux_q  InternalRulePriority=Speed  RndMeth=Simplest
      settings: InputPortMap=u0,u1
  Ldq Lookup Table : Lookup_n-D  BreakpointsForDimension1=d_current_q_Flux  BreakpointsForDimension2=q_current_q_Flux  BreakpointsForDimension3=[5, 7]  Table=Ldq  ExtrapMethod=Clip  UseLastTableValue=on  InternalRulePriority=Speed  OutDataTypeStr=Inherit: Inherit from 'Table data'  RndMeth=Simplest
      settings: InputPortMap=u0,u1
  Lqd Lookup Table1 : Lookup_n-D  BreakpointsForDimension1=d_current_q_Flux  BreakpointsForDimension2=q_current_q_Flux  BreakpointsForDimension3=[5, 7]  Table=Ldq  ExtrapMethod=Clip  UseLastTableValue=on  InternalRulePriority=Speed  OutDataTypeStr=Inherit: Inherit from 'Table data'  RndMeth=Simplest
      settings: InputPortMap=u0,u1
  Scope : Scope  NumInputPorts=4
  psi_d_set : Outport
  psi_q_set : Outport  Port=2
  psi_d_LUT : Outport  Port=3
  psi_q_LUT : Outport  Port=4
  Ldq_LUT : Outport  Port=5
  Lqd_LUT : Outport  Port=6
  wires:
  I_d_set/1 -> Scope/1, Flux_d Lookup Table1/1
  I_q_set/1 -> Scope/2, Flux_q Lookup Table2/2
  Flux_d Lookup Table1/1 -> psi_d_set/1  "psi_d_set"
  Flux_q Lookup Table2/1 -> psi_q_set/1  "psi_q_set"
  Flux_d Lookup Table/1 -> psi_d_LUT/1  "psi_d_controller"
  Flux_q Lookup Table1/1 -> psi_q_LUT/1  "psi_q_controller"
  Ldq Lookup Table/1 -> Ldq_LUT/1  "Ldq_Karte"
  Lqd Lookup Table1/1 -> Lqd_LUT/1  "Ldq_Karte"
  I_d/1 -> Scope/3, Flux_q Lookup Table2/1, Lqd Lookup Table1/1, Ldq Lookup Table/1, Flux_q Lookup Table1/1, Flux_d Lookup Table/1
  I_q/1 -> Scope/4, Lqd Lookup Table1/2, Ldq Lookup Table/2, Flux_q Lookup Table1/2, Flux_d Lookup Table1/2, Flux_d Lookup Table/2

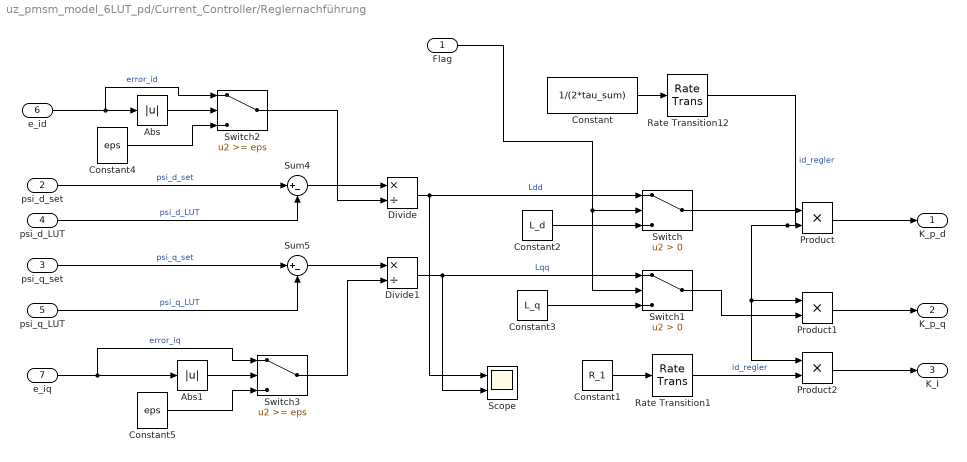
== system uz_pmsm_model_6LUT_pd/Current_Controller/Reglernachführung ==
  Flag : Inport
  psi_d_set : Inport  Port=2
  psi_q_set : Inport  Port=3
  psi_d_LUT : Inport  Port=4
  psi_q_LUT : Inport  Port=5
  e_id : Inport  Port=6
  e_iq : Inport  Port=7
  Abs : Abs  SaturateOnIntegerOverflow=off
  Abs1 : Abs  SaturateOnIntegerOverflow=off
  Constant : Constant  Value=1/(2*tau_sum)
  Constant1 : Constant  Value=R_1
  Constant2 : Constant  Value=L_d
  Constant3 : Constant  Value=L_q
  Constant4 : Constant  Value=eps  SampleTime=ts_regler
  Constant5 : Constant  Value=eps  SampleTime=ts_regler
  Divide : Product  Inputs=*/
  Divide1 : Product  Inputs=*/
  Product : Product
  Product1 : Product
  Product2 : Product
  Rate Transition1 : RateTransition  OutPortSampleTime=ts_regler
  Rate Transition12 : RateTransition  OutPortSampleTime=ts_regler
  Scope : Scope  NumInputPorts=2
  Sum4 : Sum  Inputs=|+-
  Sum5 : Sum  Inputs=|+-
  Switch : Switch  Criteria=u2 > Threshold  SaturateOnIntegerOverflow=off  InputSameDT=off
  Switch1 : Switch  Criteria=u2 > Threshold  SaturateOnIntegerOverflow=off  InputSameDT=off
  Switch2 : Switch  Threshold=eps  SaturateOnIntegerOverflow=off  InputSameDT=off
  Switch3 : Switch  Threshold=eps  SaturateOnIntegerOverflow=off  InputSameDT=off
  K_p_d : Outport
  K_p_q : Outport  Port=2
  K_I : Outport  Port=3
  wires:
  Constant/1 -> Rate Transition12/1
  Product/1 -> K_p_d/1
  Product1/1 -> K_p_q/1
  Product2/1 -> K_I/1
  Constant1/1 -> Rate Transition1/1
  Rate Transition12/1 -> Product2/1, Product1/1, Product/2  "id_regler"
  Rate Transition1/1 -> Product2/2  "id_regler"
  Flag/1 -> Switch/2, Switch1/2
  Constant2/1 -> Switch/3
  Switch/1 -> Product/1
  Constant3/1 -> Switch1/3
  Switch1/1 -> Product1/2
  Sum4/1 -> Divide/1
  psi_q_LUT/1 -> Sum5/2  "psi_q_LUT"
  Sum5/1 -> Divide1/1
  psi_d_LUT/1 -> Sum4/2  "psi_d_LUT"
  psi_d_set/1 -> Sum4/1  "psi_d_set"
  psi_q_set/1 -> Sum5/1  "psi_q_set"
  Divide/1 -> Scope/1, Switch/1  "Ldd"
  Divide1/1 -> Scope/2, Switch1/1  "Lqq"
  e_id/1 -> Switch2/1, Abs/1  "error_id"
  Constant4/1 -> Switch2/3
  Abs/1 -> Switch2/2
  Switch2/1 -> Divide/2
  e_iq/1 -> Switch3/1, Abs1/1  "error_iq"
  Switch3/1 -> Divide1/2
  Abs1/1 -> Switch3/2
  Constant5/1 -> Switch3/3

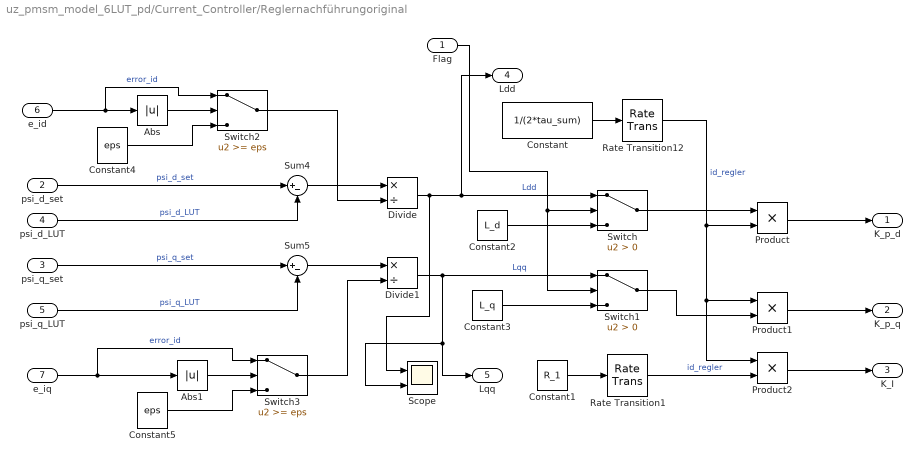
== system uz_pmsm_model_6LUT_pd/Current_Controller/Reglernachführungoriginal ==
  Flag : Inport
  psi_d_set : Inport  Port=2
  psi_q_set : Inport  Port=3
  psi_d_LUT : Inport  Port=4
  psi_q_LUT : Inport  Port=5
  e_id : Inport  Port=6
  e_iq : Inport  Port=7
  Abs : Abs  SaturateOnIntegerOverflow=off
  Abs1 : Abs  SaturateOnIntegerOverflow=off
  Constant : Constant  Value=1/(2*tau_sum)
  Constant1 : Constant  Value=R_1
  Constant2 : Constant  Value=L_d
  Constant3 : Constant  Value=L_q
  Constant4 : Constant  Value=eps  SampleTime=ts_regler
  Constant5 : Constant  Value=eps  SampleTime=ts_regler
  Divide : Product  Inputs=*/
  Divide1 : Product  Inputs=*/
  Product : Product
  Product1 : Product
  Product2 : Product
  Rate Transition1 : RateTransition  OutPortSampleTime=ts_regler
  Rate Transition12 : RateTransition  OutPortSampleTime=ts_regler
  Scope : Scope  NumInputPorts=2
  Sum4 : Sum  Inputs=|+-
  Sum5 : Sum  Inputs=|+-
  Switch : Switch  Criteria=u2 > Threshold  SaturateOnIntegerOverflow=off  InputSameDT=off
  Switch1 : Switch  Criteria=u2 > Threshold  SaturateOnIntegerOverflow=off  InputSameDT=off
  Switch2 : Switch  Threshold=eps  SaturateOnIntegerOverflow=off  InputSameDT=off
  Switch3 : Switch  Threshold=eps  SaturateOnIntegerOverflow=off  InputSameDT=off
  K_p_d : Outport
  K_p_q : Outport  Port=2
  K_I : Outport  Port=3
  Ldd : Outport  Port=4
  Lqq : Outport  Port=5
  wires:
  Constant/1 -> Rate Transition12/1
  Product/1 -> K_p_d/1
  Product1/1 -> K_p_q/1
  Product2/1 -> K_I/1
  Constant1/1 -> Rate Transition1/1
  Rate Transition12/1 -> Product2/1, Product1/1, Product/2  "id_regler"
  Rate Transition1/1 -> Product2/2  "id_regler"
  Flag/1 -> Switch/2, Switch1/2
  Constant2/1 -> Switch/3
  Switch/1 -> Product/1
  Constant3/1 -> Switch1/3
  Switch1/1 -> Product1/2
  Sum4/1 -> Divide/1
  psi_q_LUT/1 -> Sum5/2  "psi_q_LUT"
  Sum5/1 -> Divide1/1
  psi_d_LUT/1 -> Sum4/2  "psi_d_LUT"
  psi_d_set/1 -> Sum4/1  "psi_d_set"
  psi_q_set/1 -> Sum5/1  "psi_q_set"
  Divide/1 -> Scope/1, Ldd/1, Switch/1  "Ldd"
  Divide1/1 -> Scope/2, Lqq/1, Switch1/1  "Lqq"
  e_id/1 -> Switch2/1, Abs/1  "error_id"
  Constant4/1 -> Switch2/3
  Abs/1 -> Switch2/2
  Switch2/1 -> Divide/2
  e_iq/1 -> Switch3/1, Abs1/1  "error_id"
  Switch3/1 -> Divide1/2
  Abs1/1 -> Switch3/2
  Constant5/1 -> Switch3/3

== system uz_pmsm_model_6LUT_pd/uz_pmsm_model_6LUT/mechanical_system ==
  note: This delay breaks the algebraic loop between mechanical and electrical system.
      | Introduces a delay of 500ns.
  reset : Inport
  M_Mi : Inport  Port=2
  mu : Inport  Port=3
  M_n0 : Inport  Port=4
  reciprocal_J : Inport  Port=5
  load_torque : Inport  Port=6
  Abs : Abs  SaturateOnIntegerOverflow=off
  Delay : Delay  DelayLength=1
  Product11 : Product
  Product12 : Product
  Product4 : Product
  Sign1 : Signum
  Sum : Sum  Inputs=|+-  OutDataTypeStr=double
  Sum1 : Sum  Inputs=|+-
  Sum5 : Sum  Inputs=|++
  integrator1 : Subsystem
  omega_mech : Outport
  wires:
  Product11/1 -> integrator1/2(in)
  Sum5/1 -> Product4/1
  Sign1/1 -> Product4/2
  integrator1/1(outt) -> Sign1/1, Abs/1, omega_mech/1
  Abs/1 -> Product12/2
  reset/1 -> integrator1/1(reset)
  Product12/1 -> Sum5/1
  mu/1 -> Product12/1
  M_n0/1 -> Sum5/2
  reciprocal_J/1 -> Product11/1
  M_Mi/1 -> Sum/1
  Sum1/1 -> Product11/2
  load_torque/1 -> Sum1/2
  Sum/1 -> Delay/1
  Product4/1 -> Sum/2
  Delay/1 -> Sum1/1

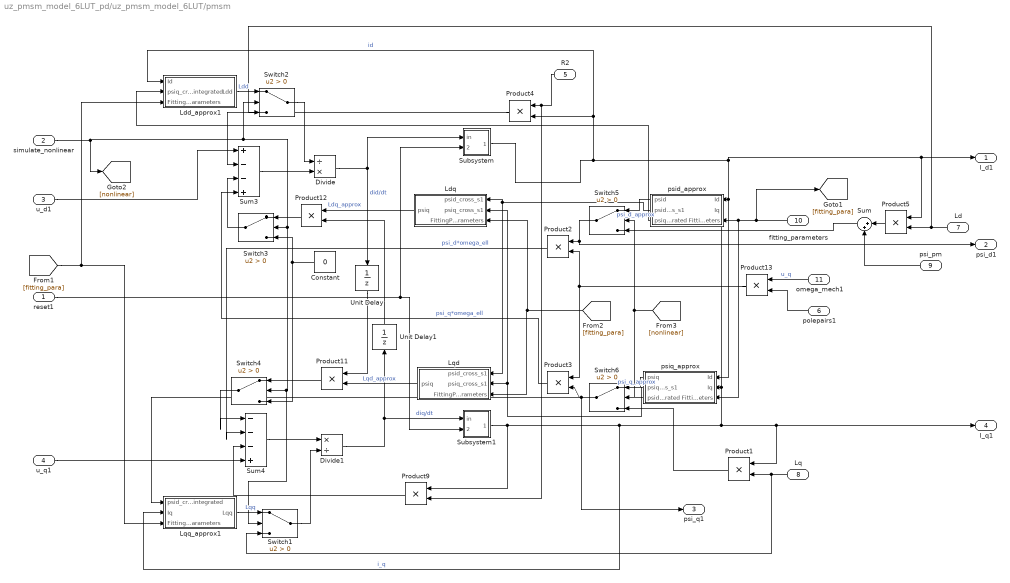
== system uz_pmsm_model_6LUT_pd/uz_pmsm_model_6LUT/pmsm ==
  reset1 : Inport
  simulate_nonlinear : Inport  Port=2
  u_d1 : Inport  Port=3
  u_q1 : Inport  Port=4
  R2 : Inport  Port=5
  polepairs1 : Inport  Port=6
  Ld : Inport  Port=7
  Lq : Inport  Port=8
  psi_pm : Inport  Port=9
  fitting_parameters : Inport  Port=10
  omega_mech1 : Inport  Port=11
  Constant : Constant  Value=0  SampleTime=ts
  Divide : Product  Inputs=/*
  Divide1 : Product  Inputs=*/  OutDataTypeStr=Inherit: Same as first input
  Ldd_approx1 : Subsystem
  Ldq : Subsystem
  Lqd : Subsystem
  Lqq_approx1 : Subsystem
  Product{1,3..5,12..13} (6 alike) : Product
  Product11 : Product  OutDataTypeStr=double
  Product2 : Product  OutDataTypeStr=double
  Product9 : Product  OutDataTypeStr=Inherit: Same as first input
  Subsystem : Subsystem
  Subsystem1 : Subsystem
  Sum : Sum  Inputs=|++
  Sum3 : Sum  Inputs=|+--+
  Sum4 : Sum  Inputs=|---+
  Switch{1..6} (6 alike) : Switch  Criteria=u2 > Threshold  SaturateOnIntegerOverflow=off  InputSameDT=off
  Unit Delay : UnitDelay  SampleTime=-1  HasFrameUpgradeWarning=on
  Unit Delay1 : UnitDelay  SampleTime=-1  HasFrameUpgradeWarning=on
  psid_approx : Subsystem
  psiq_approx : Subsystem
  I_d1 : Outport
  psi_d1 : Outport  Port=2
  psi_q1 : Outport  Port=3
  I_q1 : Outport  Port=4
  wires:
  Sum4/1 -> Divide1/1
  u_q1/1 -> Sum4/4
  Divide1/1 -> Unit Delay1/1, Subsystem1/1(in)  "diq/dt"
  polepairs1/1 -> Product13/2
  Product13/1 -> Product3/1, Product2/2
  Divide/1 -> Unit Delay/1, Subsystem/1(in)  "did/dt"
  Sum3/1 -> Divide/2
  Product9/1 -> Sum4/3
  reset1/1 -> Subsystem/2(reset), Subsystem1/2(reset)
  u_d1/1 -> Sum3/1
  R2/1 -> Product9/2, Product4/1
  Subsystem/1(outt) -> Ldd_approx1/1(Id), Product4/2, Product5/1, I_d1/1, psid_approx/1(Id), psiq_approx/1(Id)  "id"
  Subsystem1/1(outt) -> Lqq_approx1/2(Iq), I_q1/1, Product1/1, psid_approx/2(Iq), psiq_approx/2(Iq), Product9/1  "i_q"
  Product3/1 -> Sum3/4  "psi_q*omega_ell"
  Product4/1 -> Sum3/2
  Product2/1 -> Sum4/2  "psi_d*omega_ell"
  Unit Delay/1 -> Product11/1
  Unit Delay1/1 -> Product12/2
  Lqd/1(psiq) -> Product11/2  "Lqd_approx"
  Ldq/1(psiq) -> Product12/1  "Ldq_approx"
  omega_mech1/1 -> Product13/1  "u_q"
  fitting_parameters/1 -> [fitting_para], psiq_approx/3(FittingParameters), psid_approx/3(FittingParameters)
  Lqq_approx1/1(Lqq) -> Switch1/1  "Lqq"
  Switch1/1 -> Divide1/2
  Ldd_approx1/1(Ldd) -> Switch2/1  "Ldd"
  Switch2/1 -> Divide/1
  Product12/1 -> Switch3/1
  Switch3/1 -> Sum3/3
  Constant/1 -> Switch4/3, Switch3/3
  Product11/1 -> Switch4/1
  Switch4/1 -> Sum4/1
  simulate_nonlinear/1 -> Switch1/2, Switch4/2, Switch3/2, Switch2/2, [nonlinear]
  psid_approx/1(psid) -> Switch5/1  "psi_d_approx"
  Switch5/1 -> psi_d1/1, Product2/1
  Product5/1 -> Sum/1
  Ld/1 -> Switch2/3, Product5/2
  psi_pm/1 -> Sum/2
  Sum/1 -> Switch5/3
  psiq_approx/1(psiq) -> Switch6/1  "psi_q_approx"
  Switch6/1 -> psi_q1/1, Product3/2
  [nonlinear] -> Switch5/2, Switch6/2
  Lq/1 -> Switch1/3, Product1/2
  Product1/1 -> Switch6/3
  [fitting_para] -> Ldd_approx1/3(FittingParameters), Lqq_approx1/3(FittingParameters)
  [fitting_para] -> Ldq/3(FittingParameters), Lqd/3(FittingParameters)
  psiq_approx/2(psiq_cross_s1) -> Ldq/2(psiq_cross_s1), Lqd/2(psiq_cross_s1)
  psid_approx/2(psid_cross_s1) -> Ldq/1(psid_cross_s1), Lqd/1(psid_cross_s1)
  psiq_approx/3(psid_cross_s1_integrated) -> Lqq_approx1/1(psid_cross_s1_integrated)
  psid_approx/3(psiq_cross_s1_integrated) -> Ldd_approx1/2(psiq_cross_s1_integrated)

== system uz_pmsm_model_6LUT_pd/uz_pmsm_model_6LUT/torque_calculation ==
  I_d : Inport
  psi_d : Inport  Port=2
  psi_q : Inport  Port=3
  polepairs : Inport  Port=4
  I_q : Inport  Port=5
  Factor : Gain  Gain=(3/2)
  Product2 : Product
  Product3 : Product
  Product9 : Product
  Sum3 : Sum  Inputs=-|+
  M_Mi : Outport
  wires:
  Sum3/1 -> Factor/1
  Product3/1 -> Sum3/2
  Product2/1 -> Sum3/1
  psi_q/1 -> Product2/2
  psi_d/1 -> Product3/1
  I_d/1 -> Product2/1
  I_q/1 -> Product3/2
  Product9/1 -> M_Mi/1  "M_Mi"
  polepairs/1 -> Product9/2
  Factor/1 -> Product9/1  "M_Mi"

== system uz_pmsm_model_6LUT_pd/Current_Controller/Entkopplungen/Lineare_Entkopplung ==
  i_d : Inport
  i_q : Inport  Port=2
  omega_m : Inport  Port=3
  Constant1 : Constant  Value=psi_pm  SampleTime=-1
  Gain : Gain  Gain=L_q
  Gain1 : Gain  Gain=L_d
  Gain2 : Gain  Gain=polepair
  Product : Product
  Product1 : Product
  Sum6 : Sum  Inputs=|++
  u_d : Outport
  u_q : Outport  Port=2
  wires:
  omega_m/1 -> Gain2/1
  Sum6/1 -> Product1/1
  Product/1 -> u_d/1
  i_d/1 -> Gain1/1
  Constant1/1 -> Sum6/2
  i_q/1 -> Gain/1
  Product1/1 -> u_q/1
  Gain1/1 -> Sum6/1
  Gain2/1 -> Product1/2, Product/2
  Gain/1 -> Product/1

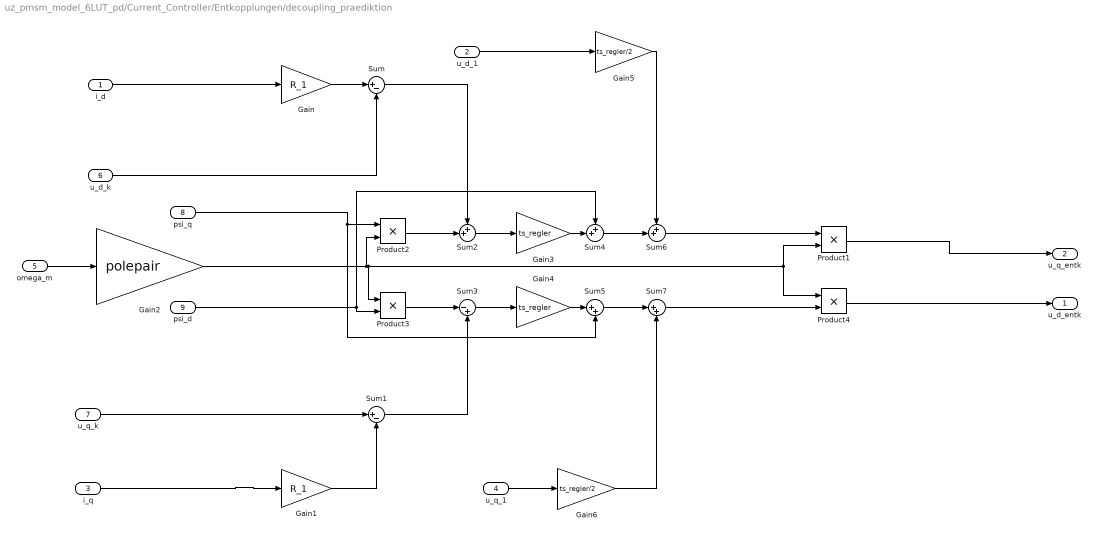
== system uz_pmsm_model_6LUT_pd/Current_Controller/Entkopplungen/decoupling_praediktion ==
  i_d : Inport
  u_d_1 : Inport  Port=2
  i_q : Inport  Port=3
  u_q_1 : Inport  Port=4
  omega_m : Inport  Port=5
  u_d_k : Inport  Port=6
  u_q_k : Inport  Port=7
  psi_q : Inport  Port=8
  psi_d : Inport  Port=9
  Gain : Gain  Gain=R_1
  Gain1 : Gain  Gain=R_1
  Gain2 : Gain  Gain=polepair
  Gain3 : Gain  Gain=ts_regler
  Gain4 : Gain  Gain=ts_regler
  Gain5 : Gain  Gain=ts_regler/2
  Gain6 : Gain  Gain=ts_regler/2
  Product{1..4} (4 alike) : Product
  Sum : Sum  Inputs=|+-
  Sum1 : Sum  Inputs=|+-
  Sum2 : Sum  Inputs=++|
  Sum3 : Sum  Inputs=|-+
  Sum4 : Sum  Inputs=++|
  Sum5 : Sum  Inputs=|++
  Sum6 : Sum  Inputs=++|
  Sum7 : Sum  Inputs=|++
  u_d_entk : Outport
  u_q_entk : Outport  Port=2
  wires:
  psi_q/1 -> Sum5/2, Product2/1
  psi_d/1 -> Product3/2, Sum4/1
  Gain2/1 -> Product1/2, Product4/1, Product3/1, Product2/2
  u_d_k/1 -> Sum/2
  Gain/1 -> Sum/1
  u_q_k/1 -> Sum1/1
  Gain1/1 -> Sum1/2
  Product3/1 -> Sum3/1
  Product2/1 -> Sum2/2
  Sum/1 -> Sum2/1
  Sum1/1 -> Sum3/2
  Sum3/1 -> Gain4/1
  Sum2/1 -> Gain3/1
  Gain3/1 -> Sum4/2
  Gain4/1 -> Sum5/1
  u_d_1/1 -> Gain5/1
  Sum4/1 -> Sum6/2
  u_q_1/1 -> Gain6/1
  Gain5/1 -> Sum6/1
  Sum5/1 -> Sum7/1
  Gain6/1 -> Sum7/2
  Sum6/1 -> Product1/1
  Sum7/1 -> Product4/2
  omega_m/1 -> Gain2/1
  i_d/1 -> Gain/1
  i_q/1 -> Gain1/1
  Product1/1 -> u_q_entk/1
  Product4/1 -> u_d_entk/1

== system uz_pmsm_model_6LUT_pd/Current_Controller/Entkopplungen/dynamic_nonlinear_entkopplung1 ==
  i_d : Inport
  i_q : Inport  Port=2
  psi_d : Inport  Port=3
  psi_q : Inport  Port=4
  Ldq_LUT : Inport  Port=5
  Lqd_LUT : Inport  Port=6
  omega_m : Inport  Port=7
  Gain2 : Gain  Gain=polepair
  Product{,1..3} (4 alike) : Product
  Sum1 : Sum  Inputs=++|
  Sum6 : Sum  Inputs=++|
  u_d : Outport
  u_q : Outport  Port=2
  wires:
  psi_q/1 -> Product/1  "psi_q_LUT"
  Gain2/1 -> Product1/2, Product/2
  psi_d/1 -> Product1/1  "psi_d_LUT"
  omega_m/1 -> Gain2/1
  i_d/1 -> Product2/1
  Ldq_LUT/1 -> Product2/2
  Sum6/1 -> u_q/1
  Product1/1 -> Sum6/2
  Product/1 -> Sum1/2
  Sum1/1 -> u_d/1
  i_q/1 -> Product3/1
  Lqd_LUT/1 -> Product3/2
  Product3/1 -> Sum6/1
  Product2/1 -> Sum1/1

== system uz_pmsm_model_6LUT_pd/Current_Controller/Entkopplungen/static_nonlinear_entkopplung ==
  psi_d : Inport
  psi_q : Inport  Port=2
  omega_m : Inport  Port=3
  Gain2 : Gain  Gain=polepair
  Product : Product
  Product1 : Product
  Scope : Scope  NumInputPorts=2
  u_d : Outport
  u_q : Outport  Port=2
  wires:
  psi_q/1 -> Product/1  "psi_q_LUT"
  Gain2/1 -> Product1/2, Product/2
  Product1/1 -> Scope/1, u_q/1
  Product/1 -> Scope/2, u_d/1
  psi_d/1 -> Product1/1  "psi_d_LUT"
  omega_m/1 -> Gain2/1

== system uz_pmsm_model_6LUT_pd/uz_pmsm_model_6LUT/mechanical_system/integrator1 ==
  reset : Inport
  in : Inport  Port=2
  Delay1 : Delay  DelayLength=1  ExternalReset=Level
      settings: InputPortMap=u0,r5
  Gain : Gain  Gain=ts  OutDataTypeStr=double
  Sum3 : Sum  Inputs=|++  OutDataTypeStr=double
  outt : Outport
  wires:
  in/1 -> Gain/1
  Gain/1 -> Sum3/1
  reset/1 -> Delay1/2
  Sum3/1 -> Delay1/1
  Delay1/1 -> Sum3/2, outt/1
